simulink model "LearjetBlocks"  (R2015b)
settings: Solver=ode1  StartTime=0.0  StopTime=inf  FixedStep=dt  RelTol=1e-3
StopFcn:
  | set(handles.pushbutton1,'String','Start');
  | set(handles.popupmenu1,'Enable','on');
  | 
  | saveData;
model workspace (MAT data in the model file):
  gBubble = Simulink.Signal
  gBubble.DataType = 'double'
  gBubble.Dimensions = 1
  gBubble.DimensionsMode = 'Fixed'
  gBubble.Complexity = 'real'
  gBubble.SampleTime = -1
  gBubble.SamplingMode = 'auto'
  gBubble.InitialValue = 'bubble'
  gFeetPerDegLonPoly = Simulink.Signal
  gFeetPerDegLonPoly.DataType = 'double'
  gFeetPerDegLonPoly.Dimensions = 4
  gFeetPerDegLonPoly.DimensionsMode = 'Fixed'
  gFeetPerDegLonPoly.Complexity = 'real'
  gFeetPerDegLonPoly.SampleTime = -1
  gFeetPerDegLonPoly.SamplingMode = 'auto'
  gFeetPerDegLonPoly.InitialValue = 'feetPerDegLonPoly'
  gGHeight = Simulink.Signal
  gGHeight.DataType = 'double'
  gGHeight.Dimensions = 1
  gGHeight.DimensionsMode = 'Fixed'
  gGHeight.Complexity = 'real'
  gGHeight.SampleTime = -1
  gGHeight.SamplingMode = 'auto'
  gGHeight.InitialValue = 'gHeight'
  gGammaLimit = Simulink.Signal
  gGammaLimit.DataType = 'double'
  gGammaLimit.Dimensions = 1
  gGammaLimit.DimensionsMode = 'Fixed'
  gGammaLimit.Complexity = 'real'
  gGammaLimit.SampleTime = -1
  gGammaLimit.SamplingMode = 'auto'
  gGammaLimit.InitialValue = 'gammaLimit'
  gM = Simulink.Signal
  gM.DataType = 'double'
  gM.Dimensions = [3 3]
  gM.DimensionsMode = 'Fixed'
  gM.Complexity = 'real'
  gM.SampleTime = -1
  gM.SamplingMode = 'auto'
  gM.InitialValue = 'M'
  gNumberOfPaths = Simulink.Signal
  gNumberOfPaths.DataType = 'double'
  gNumberOfPaths.Dimensions = 1
  gNumberOfPaths.DimensionsMode = 'Fixed'
  gNumberOfPaths.Complexity = 'real'
  gNumberOfPaths.SampleTime = -1
  gNumberOfPaths.SamplingMode = 'auto'
  gNumberOfPaths.InitialValue = 'numberOfPaths'
  gOdeDt = Simulink.Signal
  gOdeDt.DataType = 'double'
  gOdeDt.Dimensions = 1
  gOdeDt.DimensionsMode = 'Fixed'
  gOdeDt.Complexity = 'real'
  gOdeDt.SampleTime = -1
  gOdeDt.SamplingMode = 'auto'
  gOdeDt.InitialValue = 'odeDt'
  gPredictionTime = Simulink.Signal
  gPredictionTime.DataType = 'double'
  gPredictionTime.Dimensions = 1
  gPredictionTime.DimensionsMode = 'Fixed'
  gPredictionTime.Complexity = 'real'
  gPredictionTime.SampleTime = -1
  gPredictionTime.SamplingMode = 'auto'
  gPredictionTime.InitialValue = 'predictionTime'
  gPredictionTimeBuffer = Simulink.Signal
  gPredictionTimeBuffer.DataType = 'double'
  gPredictionTimeBuffer.Dimensions = 1
  gPredictionTimeBuffer.DimensionsMode = 'Fixed'
  gPredictionTimeBuffer.Complexity = 'real'
  gPredictionTimeBuffer.SampleTime = -1
  gPredictionTimeBuffer.SamplingMode = 'auto'
  gPredictionTimeBuffer.InitialValue = 'predictionTimeBuffer'
undefined symbols (not defined in the file or in its folder): dt, dtedHotMatrix, dtedLatMatrix, dtedLonMatrix, executePath, feetPerDegLatPoly, feetPerDegLonPoly, gammaLimit, odeCmdMatrixNz, odeCmdMatrixPhi, odeCmdVectorTime, odeTimeVector, origin, stopTime
libraries: simulink x3
settings Model: Creator=dev  LastModifiedBy=jay.kemper
settings DataIOCC: SaveFormat=Array
settings DebuggingCC: SolverPrmCheckMsg=warning
settings HardwareCC: ProdBitPerPointer=32  ProdLargestAtomicFloat=None  ProdIntDivRoundTo=Undefined  ProdEndianess=Unspecified  ProdWordSize=32  ProdHWDeviceType=32-bit Generic
settings ModelReferenceCC: EnableParallelModelReferenceBuilds=on
settings GRTTargetCC: GeneratePreprocessorConditionals=Disable all
settings ConfigComp: CovModelRefEnable=Off  CovSFcnEnable=off

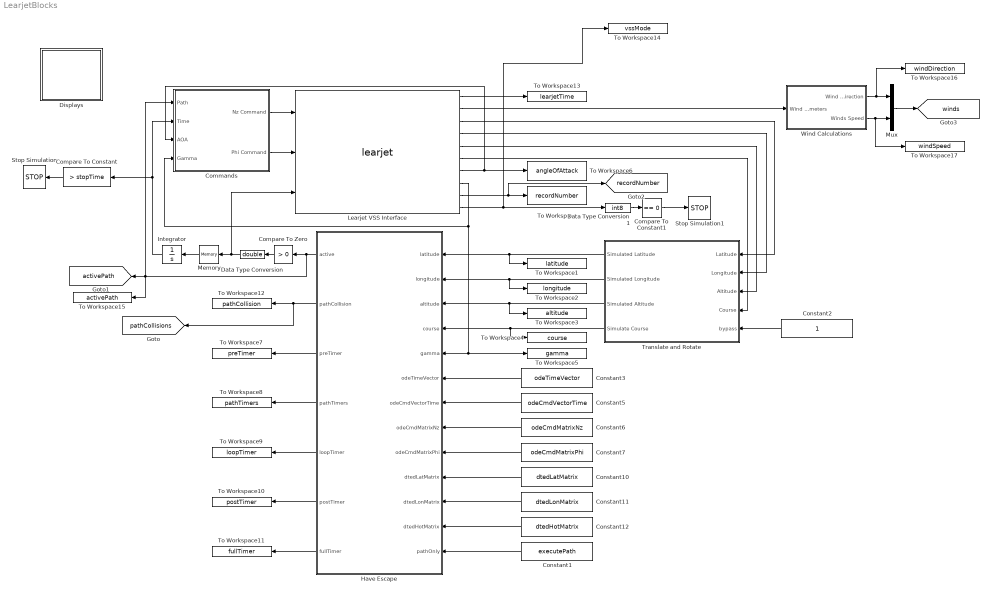
== system LearjetBlocks ==
  Commands : Subsystem
  Compare To Constant : simulink/Logic and Bit Operations/Compare To Constant  relop=>  const=stopTime  OutDataTypeStr=boolean
  Compare To Constant1 : simulink/Logic and Bit Operations/Compare To Constant  relop===  const=0  OutDataTypeStr=boolean
  Compare To Zero : simulink/Logic and Bit Operations/Compare To Zero  relop=>  OutDataTypeStr=boolean
  Constant1 : Constant  Value=executePath
  Constant10 : Constant  Value=dtedLatMatrix
  Constant11 : Constant  Value=dtedLonMatrix
  Constant12 : Constant  Value=dtedHotMatrix
  Constant2 : Constant
  Constant3 : Constant  Value=odeTimeVector
  Constant5 : Constant  Value=odeCmdVectorTime
  Constant6 : Constant  Value=odeCmdMatrixNz
  Constant7 : Constant  Value=odeCmdMatrixPhi
  Data Type Conversion : DataTypeConversion  OutDataTypeStr=double
  Data Type Conversion1 : DataTypeConversion  OutDataTypeStr=int8
  Displays : Subsystem
  Have Escape : MATLAB Function  TreatAsAtomicUnit=on
  Integrator : Integrator
  Learjet VSS Interface : S-Function  FunctionName=learjet  Parameters=target  SFunctionDeploymentMode=off  EnableBusSupport=off  mask(Learjet Ethernet Interface){target='192.168.4.11'}
      mask prompts: target "IP Address"
      mask help: This block will communicate with the Learjet VSS.
      mask Display:
      | disp(['Learjet @\n' target])
      | port_label('output',1,'Learjet Time')
      | port_label('output',2,'Wind Calculation')
      | port_label('output',3,'Latitude')
      | port_label('output',4,'Longitude')
      | port_label('output',5,'Altitude')
      | port_label('output',6,'Course')
      | port_label('output',7,'AOA')
      | port_label('output',8,'Gamma')
      | port_label('output',9,'Record Number')
      | port_label('output',10,'VSS Mode')
      | port_label('input',1,'G command')
      | port_label('input',2,'Phi command')
      | port_label('input',3,'Active')
  Memory : Memory
  Mux : Mux  Inputs=2
  Stop Simulation : Stop
  Stop Simulation1 : Stop
  To Workspace : ToWorkspace  VariableName=recordNumber  SampleTime=-1
      settings: Save2DSignal=2-D array (concatenate along first dimension)
  To Workspace1 : ToWorkspace  VariableName=latitude  SampleTime=-1
      settings: Save2DSignal=2-D array (concatenate along first dimension)
  To Workspace10 : ToWorkspace  VariableName=postTimer  SampleTime=-1
      settings: Save2DSignal=2-D array (concatenate along first dimension)
  To Workspace11 : ToWorkspace  VariableName=fullTimer  SampleTime=-1
      settings: Save2DSignal=2-D array (concatenate along first dimension)
  To Workspace12 : ToWorkspace  VariableName=pathCollision  SampleTime=-1
      settings: Save2DSignal=2-D array (concatenate along first dimension)
  To Workspace13 : ToWorkspace  VariableName=learjetTime  SampleTime=-1
      settings: Save2DSignal=2-D array (concatenate along first dimension)
  To Workspace14 : ToWorkspace  VariableName=vssMode  SampleTime=-1
      settings: Save2DSignal=2-D array (concatenate along first dimension)
  To Workspace15 : ToWorkspace  VariableName=activePath  SampleTime=-1
      settings: Save2DSignal=2-D array (concatenate along first dimension)
  To Workspace16 : ToWorkspace  VariableName=windDirection  SampleTime=-1
      settings: Save2DSignal=2-D array (concatenate along first dimension)
  To Workspace17 : ToWorkspace  VariableName=windSpeed  SampleTime=-1
      settings: Save2DSignal=2-D array (concatenate along first dimension)
  To Workspace2 : ToWorkspace  VariableName=longitude  SampleTime=-1
      settings: Save2DSignal=2-D array (concatenate along first dimension)
  To Workspace3 : ToWorkspace  VariableName=altitude  SampleTime=-1
      settings: Save2DSignal=2-D array (concatenate along first dimension)
  To Workspace4 : ToWorkspace  VariableName=course  SampleTime=-1
      settings: Save2DSignal=2-D array (concatenate along first dimension)
  To Workspace5 : ToWorkspace  VariableName=gamma  SampleTime=-1
      settings: Save2DSignal=2-D array (concatenate along first dimension)
  To Workspace6 : ToWorkspace  VariableName=angleOfAttack  SampleTime=-1
      settings: Save2DSignal=2-D array (concatenate along first dimension)
  To Workspace7 : ToWorkspace  VariableName=preTimer  SampleTime=-1
      settings: Save2DSignal=2-D array (concatenate along first dimension)
  To Workspace8 : ToWorkspace  VariableName=pathTimers  SampleTime=-1
      settings: Save2DSignal=2-D array (concatenate along first dimension)
  To Workspace9 : ToWorkspace  VariableName=loopTimer  SampleTime=-1
      settings: Save2DSignal=2-D array (concatenate along first dimension)
  Translate and Rotate : Subsystem
  Wind Calculations : Subsystem
  tag scope: activePath=global, pathCollisions=global, recordNumber=global, winds=global
  wires:
  Compare To Zero/1 -> Data Type Conversion/1
  Integrator/1 -> Commands/2(Time), Compare To Constant/1
  Memory/1 -> Integrator/1
  Translate and Rotate/1(Simulated Latitude) -> To Workspace1/1, Have Escape/1(latitude)
  Translate and Rotate/3(Simulated Altitude) -> Have Escape/3(altitude), To Workspace3/1
  Translate and Rotate/4(Simulate Course) -> Have Escape/4(course), To Workspace4/1
  Data Type Conversion/1 -> Learjet VSS Interface/3, Memory/1
  Constant2/1 -> Translate and Rotate/5(bypass)
  Compare To Constant/1 -> Stop Simulation/1
  Commands/1(Nz Command) -> Learjet VSS Interface/1
  Commands/2(Phi Command) -> Learjet VSS Interface/2
  Translate and Rotate/2(Simulated Longitude) -> To Workspace2/1, Have Escape/2(longitude)
  Constant3/1 -> Have Escape/6(odeTimeVector)
  Constant5/1 -> Have Escape/7(odeCmdVectorTime)
  Constant6/1 -> Have Escape/8(odeCmdMatrixNz)
  Constant7/1 -> Have Escape/9(odeCmdMatrixPhi)
  Constant1/1 -> Have Escape/13(pathOnly)
  Constant12/1 -> Have Escape/12(dtedHotMatrix)
  Constant10/1 -> Have Escape/10(dtedLatMatrix)
  Constant11/1 -> Have Escape/11(dtedLonMatrix)
  Have Escape/1(active) -> To Workspace15/1, Commands/1(Path), [activePath], Compare To Zero/1
  Have Escape/3(preTimer) -> To Workspace7/1
  Have Escape/5(loopTimer) -> To Workspace9/1
  Have Escape/6(postTimer) -> To Workspace10/1
  Have Escape/7(fullTimer) -> To Workspace11/1
  Have Escape/4(pathTimers) -> To Workspace8/1
  Have Escape/2(pathCollision) -> [pathCollisions], To Workspace12/1
  Learjet VSS Interface/9 -> [recordNumber], To Workspace/1
  Learjet VSS Interface/7 -> Commands/3(AOA), To Workspace6/1
  Learjet VSS Interface/8 -> Commands/4(Gamma), Have Escape/5(gamma), To Workspace5/1
  Learjet VSS Interface/6 -> Translate and Rotate/4(Course)
  Learjet VSS Interface/5 -> Translate and Rotate/3(Altitude)
  Learjet VSS Interface/4 -> Translate and Rotate/2(Longitude)
  Learjet VSS Interface/3 -> Translate and Rotate/1("Latitude ")
  Learjet VSS Interface/2 -> Wind Calculations/1(Wind Parameters)
  Learjet VSS Interface/1 -> To Workspace13/1
  Learjet VSS Interface/10 -> To Workspace14/1, Data Type Conversion1/1
  Data Type Conversion1/1 -> Compare To Constant1/1
  Wind Calculations/1(Wind Direction) -> To Workspace16/1, Mux/1
  Wind Calculations/2("Winds Speed ") -> To Workspace17/1, Mux/2
  Mux/1 -> [winds]
  Compare To Constant1/1 -> Stop Simulation1/1

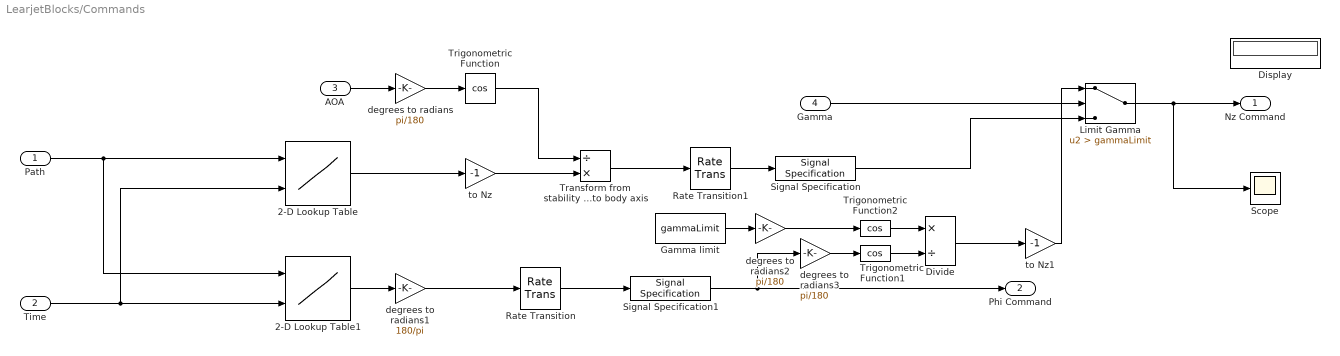
== system LearjetBlocks/Commands ==
  Path : Inport
  Time : Inport  Port=2
  AOA : Inport  Port=3
  Gamma : Inport  Port=4
  2-D Lookup Table : Lookup_n-D  BreakpointsForDimension1=[1:5]  BreakpointsForDimension2=0:.005:60  Table=cmdMatrixNz'  InternalRulePriority=Speed  RndMeth=Simplest  InputSameDT=on
  2-D Lookup Table1 : Lookup_n-D  BreakpointsForDimension1=[1:5]  BreakpointsForDimension2=0:.005:60  Table=cmdMatrixPhi'  InternalRulePriority=Speed  RndMeth=Simplest  InputSameDT=on
  Display : Display
  Divide : Product  Inputs=*/
  Gamma limit : Constant  Value=gammaLimit
  Limit Gamma : Switch  Criteria=u2 > Threshold  Threshold=gammaLimit
  Rate Transition : RateTransition
  Rate Transition1 : RateTransition
  Scope : Scope
  Signal Specification : SignalSpecification  SampleTime=dt
  Signal Specification1 : SignalSpecification  SampleTime=dt
  Transform from stability axis to body axis : Product  Inputs=/*
  Trigonometric Function : Trigonometry  Operator=cos  ApproximationMethod=CORDIC
  Trigonometric Function1 : Trigonometry  Operator=cos  ApproximationMethod=CORDIC
  Trigonometric Function2 : Trigonometry  Operator=cos  ApproximationMethod=CORDIC
  degrees to radians : Gain  Gain=pi/180
  degrees to radians1 : Gain  Gain=180/pi
  degrees to radians2 : Gain  Gain=pi/180
  degrees to radians3 : Gain  Gain=pi/180
  to Nz : Gain  Gain=-1
  to Nz1 : Gain  Gain=-1
  Nz Command : Outport
  Phi Command : Outport  Port=2
  wires:
  Path/1 -> 2-D Lookup Table1/1, 2-D Lookup Table/1
  Time/1 -> 2-D Lookup Table1/2, 2-D Lookup Table/2
  2-D Lookup Table1/1 -> degrees to radians1/1
  degrees to radians/1 -> Trigonometric Function/1
  Transform from stability axis to body axis/1 -> Rate Transition1/1
  2-D Lookup Table/1 -> to Nz/1
  to Nz/1 -> Transform from stability axis to body axis/2
  Trigonometric Function/1 -> Transform from stability axis to body axis/1
  degrees to radians1/1 -> Rate Transition/1
  Rate Transition/1 -> Signal Specification1/1
  Rate Transition1/1 -> Signal Specification/1
  Signal Specification1/1 -> degrees to radians3/1, Phi Command/1
  Limit Gamma/1 -> Scope/1, Nz Command/1
  Gamma/1 -> Limit Gamma/2
  degrees to radians3/1 -> Trigonometric Function1/1
  degrees to radians2/1 -> Trigonometric Function2/1
  Signal Specification/1 -> Limit Gamma/3
  Trigonometric Function1/1 -> Divide/2
  Trigonometric Function2/1 -> Divide/1
  Divide/1 -> to Nz1/1
  to Nz1/1 -> Limit Gamma/1
  Gamma limit/1 -> degrees to radians2/1
  AOA/1 -> degrees to radians/1

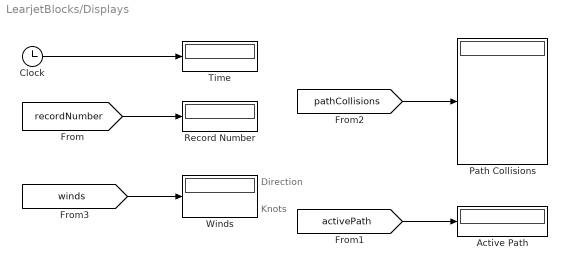
== system LearjetBlocks/Displays ==
  note: Knots
  note: Direction
  Active Path : Display
  Clock : Clock
  Path Collisions : Display
  Record Number : Display
  Time : Display
  Winds : Display
  wires:
  [recordNumber] -> Record Number/1
  [activePath] -> Active Path/1
  [pathCollisions] -> Path Collisions/1
  [winds] -> Winds/1
  Clock/1 -> Time/1

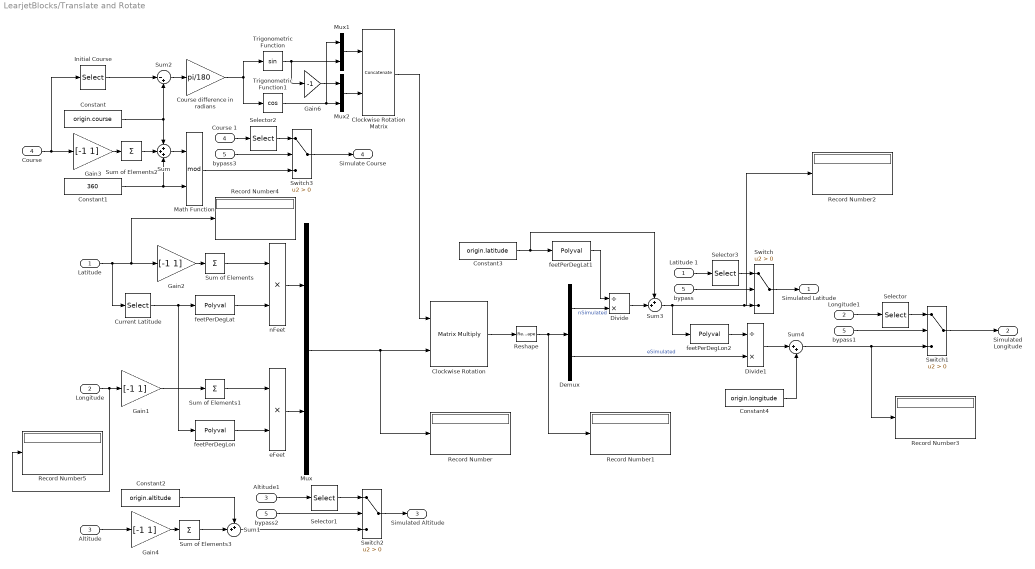
== system LearjetBlocks/Translate and Rotate ==
  "Latitude " : Inport
  Longitude : Inport  Port=2
  Altitude : Inport  Port=3
  Course : Inport  Port=4
  bypass : Inport  Port=5
  Altitude1 : InportShadow  Port=3
  Clockwise Rotation : Product  Multiplication=Matrix(*)
  Clockwise Rotation Matrix : Concatenate  Mode=Multidimensional array  ConcatenateDimension=2
  Constant : Constant  Value=origin.course
  Constant1 : Constant  Value=360
  Constant2 : Constant  Value=origin.altitude
  Constant3 : Constant  Value=origin.latitude
  Constant4 : Constant  Value=origin.longitude
  Course 1 : InportShadow  Port=4
  Course difference in radians : Gain  Gain=pi/180
  Current Latitude : Selector  InputPortWidth=2  IndexOptions=Index vector (dialog)  Indices=2  OutputSizes=1
  Demux : Demux  Outputs=2
  Divide : Product  Inputs=/*
  Divide1 : Product  Inputs=/*
  Gain{1..4} (4 alike) : Gain  Gain=[-1 1]
  Gain6 : Gain  Gain=-1
  Initial Course : Selector  InputPortWidth=2  IndexOptions=Index vector (dialog)  Indices=1  OutputSizes=1
  Latitude 1 : InportShadow
  Longitude1 : InportShadow  Port=2
  Math Function : Math  Operator=mod  SaturateOnIntegerOverflow=on
  Mux : Mux  Inputs=2
  Mux1 : Mux  Inputs=2
  Mux2 : Mux  Inputs=2
  Record Number{,1..5} (6 alike) : Display
  Reshape : Reshape
  Selector{,1..3} (4 alike) : Selector  InputPortWidth=2  IndexOptions=Index vector (dialog)  Indices=2  OutputSizes=1
  Sum : Sum  Inputs=+++
  Sum of Elements{,1..3} (4 alike) : Sum  Inputs=+
  Sum1 : Sum  Inputs=++|
  Sum2 : Sum  Inputs=|-+
  Sum3 : Sum  Inputs=++|
  Sum4 : Sum  Inputs=|++
  Switch{,1..3} (4 alike) : Switch  Criteria=u2 > Threshold
  Trigonometric Function : Trigonometry
  Trigonometric Function1 : Trigonometry  Operator=cos
  bypass1 : InportShadow  Port=5
  bypass2 : InportShadow  Port=5
  bypass3 : InportShadow  Port=5
  eFeet : Product
  feetPerDegLat : Polyval  Coefs=feetPerDegLatPoly
  feetPerDegLat1 : Polyval  Coefs=feetPerDegLatPoly
  feetPerDegLon : Polyval  Coefs=feetPerDegLonPoly
  feetPerDegLon2 : Polyval  Coefs=feetPerDegLonPoly
  nFeet : Product
  Simulated Latitude : Outport
  Simulated Longitude : Outport  Port=2
  Simulated Altitude : Outport  Port=3
  Simulate Course : Outport  Port=4
  wires:
  "Latitude "/1 -> Record Number4/1, Gain2/1, Current Latitude/1
  Gain2/1 -> Sum of Elements/1
  Current Latitude/1 -> feetPerDegLon/1, feetPerDegLat/1
  Sum of Elements/1 -> nFeet/1
  feetPerDegLat/1 -> nFeet/2
  Longitude/1 -> Record Number5/1, Gain1/1
  Gain1/1 -> Sum of Elements1/1
  Sum of Elements1/1 -> eFeet/1
  feetPerDegLon/1 -> eFeet/2
  nFeet/1 -> Mux/1
  eFeet/1 -> Mux/2
  Gain3/1 -> Sum of Elements2/1
  Course/1 -> Initial Course/1, Gain3/1
  Sum of Elements2/1 -> Sum/2
  Sum/1 -> Math Function/1
  Constant1/1 -> Sum/3, Math Function/2
  Constant/1 -> Sum/1, Sum2/2
  Gain4/1 -> Sum of Elements3/1
  Altitude/1 -> Gain4/1
  Constant2/1 -> Sum1/1
  Sum of Elements3/1 -> Sum1/2
  Initial Course/1 -> Sum2/1
  Sum2/1 -> Course difference in radians/1
  Course difference in radians/1 -> Trigonometric Function1/1, Trigonometric Function/1
  Mux1/1 -> Clockwise Rotation Matrix/1
  Mux2/1 -> Clockwise Rotation Matrix/2
  Mux/1 -> Record Number/1, Clockwise Rotation/2
  Clockwise Rotation Matrix/1 -> Clockwise Rotation/1
  Clockwise Rotation/1 -> Reshape/1
  Trigonometric Function/1 -> Mux1/2, Gain6/1
  Trigonometric Function1/1 -> Mux1/1, Mux2/2
  Reshape/1 -> Record Number1/1, Demux/1
  Demux/1 -> Divide/2  "nSimulated"
  Constant3/1 -> Sum3/1, feetPerDegLat1/1
  Constant4/1 -> Sum4/2
  Divide/1 -> Sum3/2
  Sum3/1 -> Record Number2/1, Switch/3, feetPerDegLon2/1
  feetPerDegLat1/1 -> Divide/1
  Demux/2 -> Divide1/2  "eSimulated"
  feetPerDegLon2/1 -> Divide1/1
  Divide1/1 -> Sum4/1
  Switch/1 -> Simulated Latitude/1
  bypass/1 -> Switch/2
  Sum4/1 -> Record Number3/1, Switch1/3
  bypass1/1 -> Switch1/2
  Longitude1/1 -> Selector/1
  Switch1/1 -> Simulated Longitude/1
  bypass2/1 -> Switch2/2
  Sum1/1 -> Switch2/3
  Altitude1/1 -> Selector1/1
  Switch2/1 -> Simulated Altitude/1
  Course 1/1 -> Selector2/1
  bypass3/1 -> Switch3/2
  Math Function/1 -> Switch3/3
  Switch3/1 -> Simulate Course/1
  Selector/1 -> Switch1/1
  Selector1/1 -> Switch2/1
  Selector2/1 -> Switch3/1
  Latitude 1/1 -> Selector3/1
  Selector3/1 -> Switch/1
  Gain6/1 -> Mux2/1

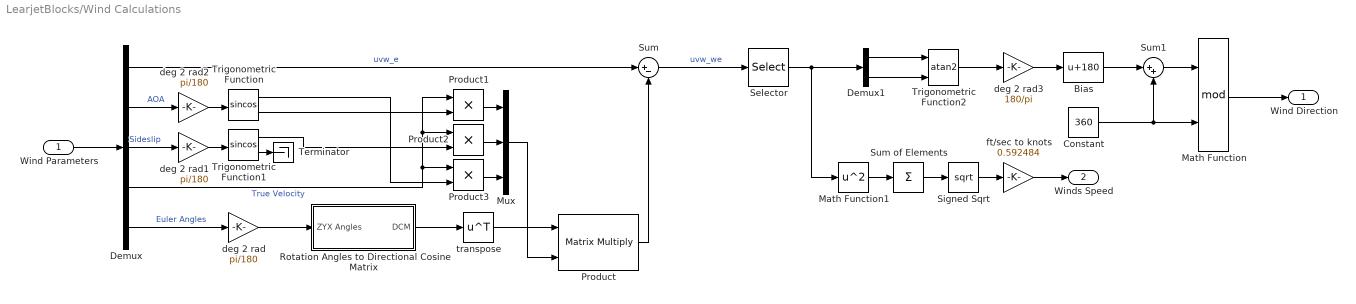
== system LearjetBlocks/Wind Calculations ==
  Wind Parameters : Inport
  Bias : Bias  Bias=180
  Constant : Constant  Value=360
  Demux : Demux  Outputs=[3 1 1 1 3]
  Demux1 : Demux  Outputs=2
  Math Function : Math  Operator=mod  SaturateOnIntegerOverflow=on
  Math Function1 : Math  Operator=square  SaturateOnIntegerOverflow=on
  Mux : Mux  Inputs=3
  Product : Product  Multiplication=Matrix(*)
  Product1 : Product
  Product2 : Product
  Product3 : Product
  Rotation Angles to Directional Cosine Matrix : Subsystem
  Selector : Selector  InputPortWidth=3  IndexOptions=Index vector (dialog)  Indices=[1 2]  OutputSizes=1
  Signed Sqrt : Sqrt  SaturateOnIntegerOverflow=on
  Sum : Sum  Inputs=|+-
  Sum of Elements : Sum  Inputs=+
  Sum1 : Sum  Inputs=|++
  Terminator : Terminator
  Trigonometric Function : Trigonometry  Operator=sincos
  Trigonometric Function1 : Trigonometry  Operator=sincos
  Trigonometric Function2 : Trigonometry  Operator=atan2  ApproximationMethod=CORDIC
  deg 2 rad : Gain  Gain=pi/180
  deg 2 rad1 : Gain  Gain=pi/180
  deg 2 rad2 : Gain  Gain=pi/180
  deg 2 rad3 : Gain  Gain=180/pi
  ft/sec to knots : Gain  Gain=0.592484
  transpose : Math  Operator=transpose  SaturateOnIntegerOverflow=on
  Wind Direction : Outport
  "Winds Speed " : Outport  Port=2
  wires:
  Wind Parameters/1 -> Demux/1
  Demux/1 -> Sum/1  "uvw_e"
  deg 2 rad/1 -> Rotation Angles to Directional Cosine Matrix/1(ZYX Angles)
  Rotation Angles to Directional Cosine Matrix/1(DCM) -> transpose/1
  transpose/1 -> Product/1
  Sum/1 -> Selector/1  "uvw_we"
  Demux/2 -> deg 2 rad2/1  "AOA"
  deg 2 rad2/1 -> Trigonometric Function/1
  Demux/3 -> deg 2 rad1/1  "Sideslip"
  Demux/5 -> deg 2 rad/1  "Euler Angles"
  Product1/1 -> Mux/1
  deg 2 rad1/1 -> Trigonometric Function1/1
  Product2/1 -> Mux/2
  Trigonometric Function/2 -> Product1/2
  Trigonometric Function1/1 -> Product2/2
  Product3/1 -> Mux/3
  Trigonometric Function/1 -> Product3/2
  Demux/4 -> Product3/1, Product1/1, Product2/1  "True Velocity"
  Mux/1 -> Product/2
  Product/1 -> Sum/2
  Trigonometric Function1/2 -> Terminator/1
  Selector/1 -> Math Function1/1, Demux1/1
  Demux1/2 -> Trigonometric Function2/2
  Demux1/1 -> Trigonometric Function2/1
  Trigonometric Function2/1 -> deg 2 rad3/1
  Sum of Elements/1 -> Signed Sqrt/1
  deg 2 rad3/1 -> Bias/1
  Sum1/1 -> Math Function/1
  Math Function/1 -> Wind Direction/1
  Bias/1 -> Sum1/1
  Constant/1 -> Math Function/2, Sum1/2
  ft/sec to knots/1 -> "Winds Speed "/1
  Math Function1/1 -> Sum of Elements/1
  Signed Sqrt/1 -> ft/sec to knots/1

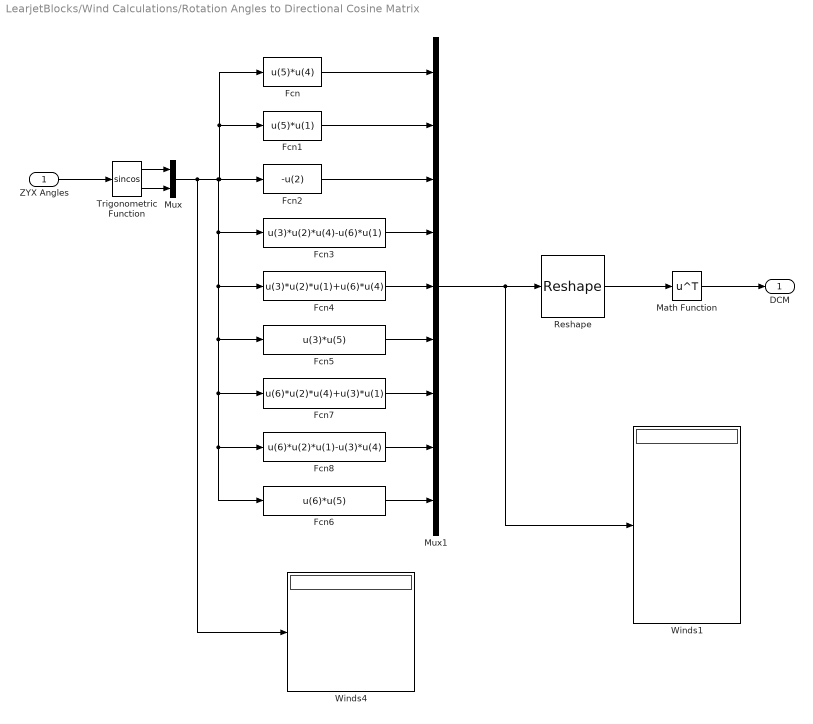
== system LearjetBlocks/Wind Calculations/Rotation Angles to Directional Cosine Matrix ==
  ZYX Angles : Inport
  Fcn : Fcn  Expr=u(5)*u(4)
  Fcn1 : Fcn  Expr=u(5)*u(1)
  Fcn2 : Fcn  Expr=-u(2)
  Fcn3 : Fcn  Expr=u(3)*u(2)*u(4)-u(6)*u(1)
  Fcn4 : Fcn  Expr=u(3)*u(2)*u(1)+u(6)*u(4)
  Fcn5 : Fcn  Expr=u(3)*u(5)
  Fcn6 : Fcn  Expr=u(6)*u(5)
  Fcn7 : Fcn  Expr=u(6)*u(2)*u(4)+u(3)*u(1)
  Fcn8 : Fcn  Expr=u(6)*u(2)*u(1)-u(3)*u(4)
  Math Function : Math  Operator=transpose  SaturateOnIntegerOverflow=on
  Mux : Mux  Inputs=2
  Mux1 : Mux  Inputs=9
  Reshape : Reshape  OutputDimensionality=Customize  OutputDimensions=[3,3]
  Trigonometric Function : Trigonometry  Operator=sincos
  Winds1 : Display
  Winds4 : Display
  DCM : Outport
  wires:
  ZYX Angles/1 -> Trigonometric Function/1
  Trigonometric Function/2 -> Mux/2
  Trigonometric Function/1 -> Mux/1
  Mux/1 -> Winds4/1, Fcn6/1, Fcn8/1, Fcn7/1, Fcn5/1, Fcn4/1, Fcn3/1, Fcn/1, Fcn1/1, Fcn2/1
  Fcn6/1 -> Mux1/9
  Fcn8/1 -> Mux1/8
  Fcn7/1 -> Mux1/7
  Fcn3/1 -> Mux1/4
  Fcn4/1 -> Mux1/5
  Fcn5/1 -> Mux1/6
  Fcn/1 -> Mux1/1
  Fcn1/1 -> Mux1/2
  Fcn2/1 -> Mux1/3
  Mux1/1 -> Winds1/1, Reshape/1
  Reshape/1 -> Math Function/1
  Math Function/1 -> DCM/1

== matlab function LearjetBlocks/Have Escape ==
  data: active output; pathCollision output; preTimer output; pathTimers output; loopTimer output; postTimer output; latitude input; longitude input; altitude input; course input; gamma input; odeTimeVector input; gPredictionTime data_store_memory; gPredictionTimeBuffer data_store_memory; gOdeDt data_store_memory; gNumberOfPaths data_store_memory; gFeetPerDegLonPoly data_store_memory; odeCmdVectorTime input; odeCmdMatrixNz input; odeCmdMatrixPhi input; dtedLatMatrix input; dtedLonMatrix input; dtedHotMatrix input; gBubble data_store_memory; gM data_store_memory; pathOnly input; fullTimer output double size=1; gGHeight data_store_memory; gGammaLimit data_store_memory
function [active,pathCollision,preTimer,pathTimers,loopTimer,postTimer,fullTimer] = HaveEscape(...
    latitude, longitude, altitude, course, gamma ...
    ,odeTimeVector,odeCmdVectorTime,odeCmdMatrixNz,odeCmdMatrixPhi ...
    ,dtedLatMatrix,dtedLonMatrix,dtedHotMatrix ...
    ,pathOnly)
%#codegen

persistent pActivePath;
persistent pPathCollisionVector;

if isempty(pActivePath) 
    pActivePath = 0;
end

if isempty(pPathCollisionVector)
    pPathCollisionVector=zeros(5,1);
end

if ( pathOnly > 0 && pathOnly <=5)
    pActivePath = pathOnly;
end

if ( pActivePath > 0 && pActivePath <=5 )
    active = pActivePath;
    fullTimer = 0;
    preTimer = 0;
    pathTimers = zeros(5,1);
    loopTimer = 0;
    postTimer = 0;
    pathCollision = pPathCollisionVector;
    return;
end

coder.extrinsic('tic');
coder.extrinsic('toc');
fullTic = uint64(zeros);
fullTic = tic;




V=523.22;                       %Constant Velocity, ft/s (310 kts)
altitudeM = ft2m(altitude);               %MSL Altitude as read from Altimeter (ft)
%%%%%%%%%%%%%%%%%%%%%%%%%%%%%%%%%%%%%%%%%%%%%%%%%%%%%%%%%%%%%%%%%%%%%%%%%%

%%%%%%%%%%%%%%%%%%%No User Inputs Below This Line%%%%%%%%%%%%%%%%%%%%%%%%%%

global gGHeight;

altitudeM = altitudeM + gGHeight;           %Current WGS-84 HAE A/C Altitude (m)

dtedLatVector = dtedLatMatrix(:,1);
dtedLonVector = dtedLonMatrix(1,:)';

hot0 = interp2(dtedLatVector,dtedLonVector,dtedHotMatrix',...
    latitude,longitude);

% if ~isfinite(hot0)
%     hot0 = altitudeM;
% end

[xM,yM,zM] = my_geodetic2enu(...
    latitude,longitude,altitudeM,...
    latitude,longitude,hot0);


% Initialize A/C state values for Propagation with ODE45
xFt = m2ft(xM);     % Initial x position, ft
yFt = m2ft(yM);     % Initial y position, ft
zFt = m2ft(zM);     % Initial z position, ft (Altitude)
%chiDeg = compass2pol(headingAngleDeg);    % Initial heading angle
coder.extrinsic('wrapTo360');
chiDeg = zeros;
chiDeg = wrapTo360(90-course);

%Initial conditions column vector [x;y;z;gam;chi] [ft,ft,ft,deg,deg]
initialConditions= [xFt;yFt;zFt;deg2rad(gamma);deg2rad(chiDeg)];

global gNumberOfPaths;
global gFeetPerDegLonPoly;

if gNumberOfPaths > 5
    gNumberOfPaths = 5;
end

% Allocate the result
% numberOfPaths = gNumberOfPaths;
% assert(odeCmdTimeLength < 1000);
% assert(numberOfPaths<6);
% aircraftProjectedPositionM = zeros(...
%     odeCmdTimeLength,...
%     3,...
%     numberOfPaths...
%     );

% Allocate result
pathCollisionVector = zeros(5,1);
pathTimerTemp = zeros(5,1);

global gBubble;
global gM;
global gPredictionTimeBuffer;

preTimer = zeros;
preTimer = toc(fullTic);

loopTic = uint64(zeros);
loopTic = tic;

for i=1:gNumberOfPaths
    
    pathTic = uint64(zeros);
    pathTic = tic;

    
    [state] = myOde( ...
        odeTimeVector,...
        initialConditions,...
        gPredictionTimeBuffer,...
        [odeCmdVectorTime odeCmdMatrixNz(:,i)],...
        [odeCmdVectorTime -odeCmdMatrixPhi(:,i)],...
        V );
    
    aircraftProjectedPositionM = ft2m(state(:,1:3));
    
% end
% 
% for i=1:gNumberOfPaths
    
    %Convert propagated position back into Lat and Lon
    [pathVectorLatDeg,pathVectorLonDeg,pathVectorAlt]=my_enu2geodetic(...
        aircraftProjectedPositionM(:,1),aircraftProjectedPositionM(:,2),aircraftProjectedPositionM(:,3),...
        latitude, longitude,hot0);
    %pathLatVectorRad=rad2deg(pathLatVectorDeg);
    %pathLonVectorRad=rad2deg(pathLonVectorDeg);
    
    
    
    
    % Logic to check the solution for terrain collision
    minDistanceBetweenAircraftAndTerrainM = zeros(1,length(odeTimeVector));
    for j=1:length(odeTimeVector)
        
        %Finds the distance between a deg of longitude at a specific Lat in km
        kmPerDegLon = ft2m(polyval(gFeetPerDegLonPoly,pathVectorLatDeg(j)))/1000;
        
        %Conversion from km to degrees for longitude distance
        bubbleRadiusinDegLon = inv(kmPerDegLon)*inv(3280.84)*gBubble; %deg Long at Lat position
        bubbleRadiusinDegLat = km2deg(gBubble);
        
        %finds the column indices Longitude DTED Posts
        dtedIndicesWithinBubbleLon=find( dtedLonVector <= (pathVectorLonDeg(j)+bubbleRadiusinDegLon)...
                                       & dtedLonVector >= (pathVectorLonDeg(j)-bubbleRadiusinDegLon) );
        
        %Finds the row indices Latitude DTED Posts
        dtedIndicesWithinBubbleLat=find( dtedLatVector <= (pathVectorLatDeg(j)+bubbleRadiusinDegLat)...
                                       & dtedLatVector >= (pathVectorLatDeg(j)-bubbleRadiusinDegLat) );
        
        %Breaks current loop iteration if no DTED Posts found
        if isempty(dtedIndicesWithinBubbleLon)==1 || isempty(dtedIndicesWithinBubbleLat)==1
            minDistanceBetweenAircraftAndTerrainM(j) = 8888;
            continue
        end
        
        
        %Finds Long/Lat values from complete Long/Lat Matrices
        localDtedLonMatrix = dtedLonMatrix(dtedIndicesWithinBubbleLat,dtedIndicesWithinBubbleLon);
        localDtedLatMatrix = dtedLatMatrix(dtedIndicesWithinBubbleLat,dtedIndicesWithinBubbleLon);
        localDtedHotMatrix = dtedHotMatrix(dtedIndicesWithinBubbleLat,dtedIndicesWithinBubbleLon); %(long,lat) because Zgrid is transposed
        
        %Build lat_lon_alt DTED posts for this timestep
        kount = numel(localDtedLonMatrix);
        assert(kount<722);
        localDtedPostList = zeros(kount,3);            
        for k=1:kount
            localDtedPostList(k,1:3)=[localDtedLatMatrix(k),localDtedLonMatrix(k),localDtedHotMatrix(k)];
        end
        
        %convert DTED to ENU
        [x,y,z]=my_geodetic2enu(...
            localDtedPostList(:,1),localDtedPostList(:,2),localDtedPostList(:,3),...
            latitude, longitude, hot0);
            %Answer in meters
        
        %Build matrices required to check if DTED are inside bubble
        dtedPostPositionMatrixM = [x,y,z];
        
        %Checks if DTED Post height is inside sphere XMX'
        xyzDtedPostBubbleOverlayLength = length(x);
        assert(xyzDtedPostBubbleOverlayLength<100);
        aircraftDistanceToDtedPost = zeros(xyzDtedPostBubbleOverlayLength,1);
        for k=1:xyzDtedPostBubbleOverlayLength
            aircraftDistanceToDtedPost(k) = ...
                (dtedPostPositionMatrixM(k,:)- aircraftProjectedPositionM(j,:))...
               *gM...
               *(dtedPostPositionMatrixM(k,:)- aircraftProjectedPositionM(j,:))';
        end
        
        %Finds the smallest distance for a given timestep
        minDistanceBetweenAircraftAndTerrainM(j) = min(aircraftDistanceToDtedPost);
    end
    
    indexOfGroundCollisions = find(minDistanceBetweenAircraftAndTerrainM <=1);
    
    %Calculates the fwd time of a collision occurring.
    
    if isempty(indexOfGroundCollisions) == 0 %Meaning: not empty
        timeOfFirstGroundCollision = odeTimeVector(indexOfGroundCollisions(1));
        pathCollisionVector(i) = timeOfFirstGroundCollision(1);
    else
        %Fills an empty matrix with -1 to delineate that no collision occured
        pathCollisionVector(i) = -1;
    end
    
    pathTimerTemp(i) = toc(pathTic);
    
end

loopTimer = zeros;
loopTimer = toc(loopTic);



    postTic = uint64(zeros);
    postTic = tic;
    
% 
% pathCollision = pPathCollisionVector;
% 


% All paths collide
if isempty(find(pathCollisionVector<0,1))
    % Look at the last collision vector
%     clearPaths = find(pPathCollisionVector<0);
%     pActivePath = clearPaths(1);
    
    % OR
    
    % Pick the largest
    largest = find(pathCollisionVector==max(pathCollisionVector));
    pActivePath = largest(1);
end


% switch length(find(pathCollisionVector<0))
%     case 0 % If all paths collide
%         pActivePath = 3; % Pick LARGEST
%     case 1 % If one escape route
%         temp = find(pathCollisionVector<0);
%         pActivePath = temp(1);
% end

pPathCollisionVector =   pathCollisionVector;
pathCollision = pPathCollisionVector;


% if all(pathCollisionVector(:) >= 0)
%     if t_grnd_col_fwd >= t_grnd_col_lft && t_grnd_col_fwd >= t_grnd_col_rgt...
%             && t_grnd_col_fwd >= t_grnd_col_lft_up && t_grnd_col_fwd >= t_grnd_col_rgt_up
%         pActivePath = 1;
%     elseif t_grnd_col_lft > t_grnd_col_fwd && t_grnd_col_lft > t_grnd_col_rgt...
%             && t_grnd_col_lft > t_grnd_col_lft_up && t_grnd_col_lft > t_grnd_col_rgt_up
%         pActivePath = 2;
%     elseif t_grnd_col_rgt > t_grnd_col_fwd && t_grnd_col_rgt > t_grnd_col_lft...
%             && t_grnd_col_rgt > t_grnd_col_lft_up && t_grnd_col_rgt > t_grnd_col_rgt_up
%         pActivePath = 3;
%     elseif t_grnd_col_lft_up > t_grnd_col_fwd && t_grnd_col_lft_up >= t_grnd_col_rgt...
%             && t_grnd_col_lft_up >= t_grnd_col_lft && t_grnd_col_lft_up >= t_grnd_col_rgt_up
%         pActivePath = 4;
%     elseif t_grnd_col_rgt_up > t_grnd_col_fwd && t_grnd_col_rgt_up >= t_grnd_col_rgt...
%             && t_grnd_col_rgt_up >= t_grnd_col_lft && t_grnd_col_rgt_up > t_grnd_col_lft_up
%         pActivePath = 5;
%     end
% end
% 

active = pActivePath;

fullTimer = zeros;
fullTimer = toc(fullTic);

postTimer = zeros;
postTimer = toc(postTic);



pathTimers = pathTimerTemp;
